simulink model "EE498_rafetkavak_termproject_part1_platooning_controlsystemdesign_simulinkmodel2"  (R2019b)
settings: Solver=VariableStepAuto  StartTime=0.0  StopTime=10  RelTol=1e-3
libraries: simulink x2
settings Model: Creator=rafet  LastModifiedBy=rafet

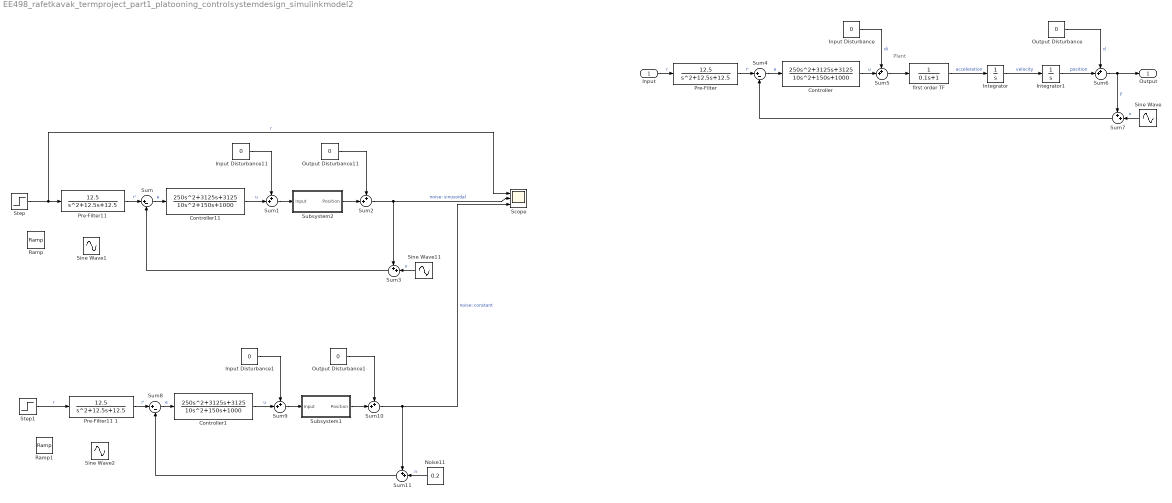
== system EE498_rafetkavak_termproject_part1_platooning_controlsystemdesign_simulinkmodel2 ==
  note: Plant
  Input : Inport
  Controller : TransferFcn  Numerator=[250 3125 3125]  Denominator=[10 150 1000]
  Controller1 : TransferFcn  Numerator=[250 3125 3125]  Denominator=[10 150 1000]
  Controller11 : TransferFcn  Numerator=[250 3125 3125]  Denominator=[10 150 1000]
  Input Disturbance : Constant  Value=0
  Input Disturbance1 : Constant  Value=0
  Input Disturbance11 : Constant  Value=0
  Integrator : Integrator
  Integrator1 : Integrator
  Noise11 : Constant  Value=0.2
  Output Disturbance : Constant  Value=0
  Output Disturbance1 : Constant  Value=0
  Output Disturbance11 : Constant  Value=0
  Pre-Filter : TransferFcn  Numerator=[12.5]  Denominator=[1 12.5 12.5]
  "Pre-Filter11 " : TransferFcn  Numerator=[12.5]  Denominator=[1 12.5 12.5]
  Pre-Filter11 1 : TransferFcn  Numerator=[12.5]  Denominator=[1 12.5 12.5]
  Ramp : simulink/Sources/Ramp  slope=1  start=0  InitialOutput=0
  Ramp1 : simulink/Sources/Ramp  slope=1  start=0  InitialOutput=0
  Scope : Scope  NumInputPorts=3
  Sine Wave : Sin  Frequency=100  SampleTime=0
  Sine Wave1 : Sin  Frequency=0.1  SampleTime=0
  Sine Wave11 : Sin  Frequency=100  SampleTime=0
  Sine Wave2 : Sin  Frequency=0.1  SampleTime=0
  Step : Step  SampleTime=0
  Step1 : Step  SampleTime=0
  Subsystem1 : Subsystem
  Subsystem2 : Subsystem
  Sum : Sum  Inputs=|+-
  Sum{1..3,5..7,9..11} (9 alike) : Sum  Inputs=++|
  Sum4 : Sum  Inputs=|+-
  Sum8 : Sum  Inputs=|+-
  first order TF : TransferFcn  Denominator=[0.1 1]
  Output : Outport
  wires:
  Sum/1 -> Controller11/1  "e"
  Controller11/1 -> Sum1/2  "u"
  Sum2/1 -> Scope/2, Sum3/1  "noise: sinusoidal"
  Sum3/1 -> Sum/2
  Sine Wave11/1 -> Sum3/2  "n"
  Output Disturbance11/1 -> Sum2/1
  Input Disturbance11/1 -> Sum1/1
  Sum1/1 -> Subsystem2/1(Input)
  Subsystem2/1(Position) -> Sum2/2
  Step/1 -> "Pre-Filter11 "/1, Scope/1  "r"
  Sine Wave/1 -> Sum7/2  "n"
  Pre-Filter/1 -> Sum4/1  "r'"
  Integrator1/1 -> Sum6/2  "position"
  Input Disturbance/1 -> Sum5/1  "di"
  Output Disturbance/1 -> Sum6/1  "d"
  Sum6/1 -> Output/1, Sum7/1  "y"
  Sum7/1 -> Sum4/2
  Sum4/1 -> Controller/1  "e"
  Input/1 -> Pre-Filter/1  "r"
  Controller/1 -> Sum5/2  "u"
  first order TF/1 -> Integrator/1  "acceleration"
  Integrator/1 -> Integrator1/1  "velocity"
  Sum5/1 -> first order TF/1
  "Pre-Filter11 "/1 -> Sum/1  "r'"
  Sum9/1 -> Subsystem1/1(Input)
  Subsystem1/1(Position) -> Sum10/2
  Input Disturbance1/1 -> Sum9/1
  Output Disturbance1/1 -> Sum10/1
  Sum10/1 -> Scope/3, Sum11/1  "noise: constant"
  Sum11/1 -> Sum8/2
  Noise11/1 -> Sum11/2  "n"
  Pre-Filter11 1/1 -> Sum8/1  "r'"
  Step1/1 -> Pre-Filter11 1/1  "r"
  Sum8/1 -> Controller1/1  "e"
  Controller1/1 -> Sum9/2  "u"

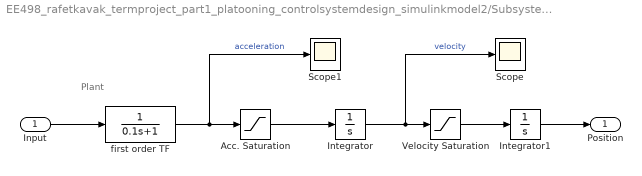
== system EE498_rafetkavak_termproject_part1_platooning_controlsystemdesign_simulinkmodel2/Subsystem1 ==
  note: Plant
  Input : Inport
  Acc. Saturation : Saturate  UpperLimit=100  LowerLimit=-100
  Integrator : Integrator
  Integrator1 : Integrator
  Scope : Scope
  Scope1 : Scope
  Velocity Saturation : Saturate  UpperLimit=100  LowerLimit=-100
  first order TF : TransferFcn  Denominator=[0.1 1]
  Position : Outport
  wires:
  Input/1 -> first order TF/1
  Integrator1/1 -> Position/1
  Integrator/1 -> Velocity Saturation/1, Scope/1  "velocity"
  Acc. Saturation/1 -> Integrator/1
  first order TF/1 -> Scope1/1, Acc. Saturation/1  "acceleration"
  Velocity Saturation/1 -> Integrator1/1

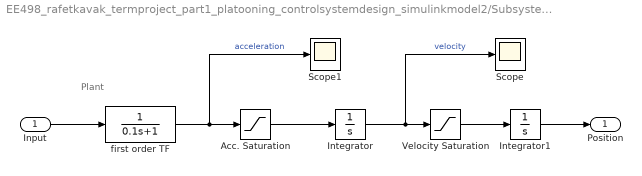
== system EE498_rafetkavak_termproject_part1_platooning_controlsystemdesign_simulinkmodel2/Subsystem2 ==
  note: Plant
  Input : Inport
  Acc. Saturation : Saturate  UpperLimit=100  LowerLimit=-100
  Integrator : Integrator
  Integrator1 : Integrator
  Scope : Scope
  Scope1 : Scope
  Velocity Saturation : Saturate  UpperLimit=100  LowerLimit=-100
  first order TF : TransferFcn  Denominator=[0.1 1]
  Position : Outport
  wires:
  Input/1 -> first order TF/1
  Integrator1/1 -> Position/1
  Integrator/1 -> Velocity Saturation/1, Scope/1  "velocity"
  Acc. Saturation/1 -> Integrator/1
  first order TF/1 -> Scope1/1, Acc. Saturation/1  "acceleration"
  Velocity Saturation/1 -> Integrator1/1
